simulink model "BoatLibraryTest01"  (R2013b)
settings: Solver=ode45  StartTime=0.0  StopTime=10  RelTol=1e-3
values from neighbouring files (symbols this model uses):
  C = C0    [Minimizer.m]    (also in parameters2.m = [1 0 0 0 0 0;0 0 1 0 0 0;0 0 0 0 1 0]; parameters3.m = [1 0 0 0 0 0;0 0 1 0 0 0;0 0 0 0 1 0])
  fw = 4    [parameters2.m]    (also in parameters3.m)
  I = 1/12*M*((2*rx1)^2 + (2*ry1)^2)    (= 7.46230507536)    [BoatController.m]    (also in boatDynamics.m; parameters2.m = 20; parameters3.m)
  inputBound = [minInput maxInput]    [parameters3.m]
  kr = 2    [parameters2.m]    (also in parameters3.m)
  M = 80*lbtokg    (= 36.28736)    [BoatController.m]    (also in parameters2.m = 10; parameters3.m)
  rx1 = -12*intom    (= -0.3048)    [BoatController.m]    (also in boatDynamics.m; costfunction.m; parameters3.m)
  rx2 = 12*intom    (= 0.3048)    [BoatController.m]    (also in boatDynamics.m; costfunction.m; parameters3.m)
  ry1 = -69*intom/2 + 6*intom    (= -0.7239)    [BoatController.m]    (also in boatDynamics.m; costfunction.m; parameters3.m)
  ry2 = ry1    (= -0.7239)    [BoatController.m]    (also in boatDynamics.m; costfunction.m; parameters3.m)
undefined symbols (not defined in the file): K
libraries: simulink x9
(part 2 of 2)

== matlab function BoatLibraryTest01/Minimizer0.2/MATLAB Function1 ==
  data: Fx input; fx output; Fy input; M input; fy output; m output; phi input
function [fx,fy,m] = fcn(Fx,Fy,M, phi)
%#codegen

R = [cosd(phi) -sin(phi) 0;...
        sind(phi)  cos(phi) 0;...
        0           0       1];
    
    FxyM = R*[Fx;Fy;M];
    
    fx = FxyM(1);
    fy = FxyM(2);
    m = FxyM(3);
    
end

== matlab function BoatLibraryTest01/MATLAB Function1 ==
  data: Fx input; y output; Fy input; M input
function y = fcn(Fx,Fy,M)
%#codegen

y = [Fx;Fy;M];

== matlab function BoatLibraryTest01/boat dynamics input [fx;fy;moment]1/MATLAB Function ==
  data: C input; x output; M input; I input; fw input; kr input; x0 input; fx input; y output; fy input; m input
function [x,y] = systemstep(C,M,I,fw,kr,x0,fx,fy,m)

   % status vector y=[x;x_dot;y;_y_dot;theta;theta_dot]
   % forces u=[fx;fy;m]
   % contant parameters {mass; rotational inertia; friction coefficients }
   
   x1 = x0(2);
   x2 = fx/M - 0*x0(2)*fw;
   x3 = x0(4);
   x4 = fy/M - 0*x0(4)*fw;
   x5 = x0(6);
   x6 = m/I - 0*x0(6)*kr;

   x=[x1;x2;x3;x4;x5;x6];
   
   y = C*x0;
